simulink model "mpc555rt_io"  (Simulink 6.0)
settings: Solver=FixedStepDiscrete  StartTime=0.0  StopTime=inf  FixedStep=0.01  RelTol=1e-3
PreLoadFcn:
  | RTWConfigurationCB('preloadfcn', bdroot);
undefined symbols (not defined in the file or in its folder): Target_IO, Target_IO_lib5
libraries: mpc555drivers x15, canblocks x8, mpc555toucan x8
CloseFcn:
  | rtwprivate ssgencode ModelCloseRequest mpc555iodemo
settings Model: Creator=The MathWorks Inc.  LastModifiedBy=batserve  ExtModeAutoUpdateStatusClock=off  ProdHWDeviceType=Motorola PowerPC
settings DataIOCC: SaveFormat=StructureWithTime  SignalLoggingName=sigsOut
settings OptimizationCC: BooleanDataType=off  InlineParams=on  InlineInvariantSignals=off  RollThreshold=10  OptimizeModelRefInitCode=on  LifeSpan=1
settings DebuggingCC: CheckExecutionContextPreStartOutputMsg=on  CheckExecutionContextRuntimeOutputMsg=on  SolverPrmCheckMsg=none
settings HardwareCC: ProdEndianess=BigEndian  ProdHWDeviceType=Motorola PowerPC  TargetHWDeviceType=32-bit Generic
settings ModelReferenceCC: UpdateModelReferenceTargets=IfOutOfDate
settings RTWCC: SystemTargetFile=mpc555rt.tlc  TemplateMakefile=mpc555rt.tmf  Description=Embedded Target for Motorola MPC555 (real-time target)  ProcessScript=mpc555rt_make_rtw_hook
settings CodeAppCC: IgnoreCustomStorageClasses=off
settings STFCustomTargetCC: TargetFcnLib=ansi_tfl_tmw.mat  GenFloatMathFcnCalls=ANSI_C  ModelReferenceCompliant=off  CombineOutputUpdateFcns=on  ERTCustomFileBanners=on  SystemTargetFile=mpc555rt.tlc
settings ERTTargetCC: TargetFcnLib=ansi_tfl_tmw.mat  GenFloatMathFcnCalls=ANSI_C  ModelReferenceCompliant=off  SupportContinuousTime=on  SupportNonInlinedSFcns=on  RootIOFormat=Individual Arguments  ERTCustomFileTemplate=example_file_process.tlc  InitialValueSource=Model
settings CustomProperty: DataType=RTWOptions_EnumType__toolbox_rtw_targets_mpc555dk_mpc555dk_mpc555rt_MPC555_OPTIMIZATION_SWITCH  Value=speed
settings EnumStrPairs: String=speed

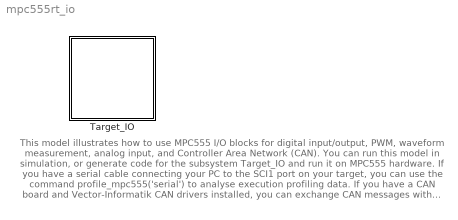
== system mpc555rt_io ==
  note: This model illustrates how to use MPC555 I/O
      | blocks for digital input/output, PWM, waveform
      | measurement, analog input, and Controller Area Network (CAN).
      |
      | You can run this model in simulation, or generate
      | code for the subsystem Target_IO and run it on
      | MPC555 hardware.
      |
      | If you have a serial cable connecting your PC to the SCI1
      | port on your target, you can use the command
      | profile_mpc555('serial') to analyse execution profiling data.
      |
      | If you have a CAN board and Vector-Informatik
      | CAN drivers installed, you can exchange CAN messages
      | with the companion model mpc555rt_iohost.
  Target_IO : Subsystem  InitFcn=|  PropExecContextAcrossSSBoundary=on
      | % START RTW CONFIGURATION CODE %
      | RTWConfigurationCB('rtw_target_initfcn',gcb);
      | % END RTW CONFIGURATION CODE %
      mask Display: image(imread('target_affordance_icon.jpg'),'bottom-right')

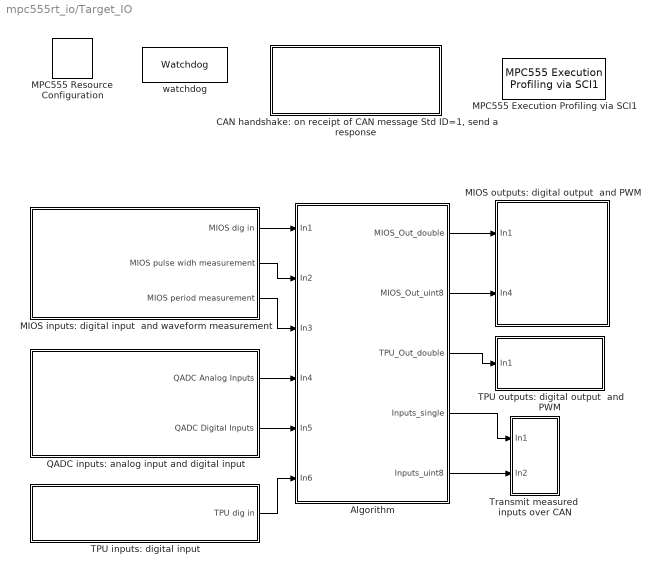
== system mpc555rt_io/Target_IO ==
  Algorithm : Subsystem  PropExecContextAcrossSSBoundary=on
  "CAN handshake: on receipt of CAN message Std ID=1, send a response" : Subsystem  PropExecContextAcrossSSBoundary=on
  MIOS inputs: digital input  and waveform measurement : Subsystem  PropExecContextAcrossSSBoundary=on
  MIOS outputs: digital output  and PWM : Subsystem  PropExecContextAcrossSSBoundary=on
  "MPC555 Resource Configuration " : mpc555drivers/MPC555 Resource Configuration  Tag=RTW CONFIGURATION BLOCK  Priority=-100000  oldParentName=Target_IO_lib5/Target_IO  oldBlockName=|  defaultConfigLibrary=mpc555drivers
      | Target_IO_lib5/Target_IO/MPC555
      | Resource
      | Configuration
  MPC555 Execution Profiling via SCI1 : mpc555drivers/Execution Profiling/MPC555 Execution Profiling via SCI1  t=0.01  execCopyFcn=off
  QADC inputs: analog input and digital input : Subsystem  PropExecContextAcrossSSBoundary=on
  TPU inputs: digital input : Subsystem  PropExecContextAcrossSSBoundary=on
  TPU outputs: digital output  and PWM : Subsystem  PropExecContextAcrossSSBoundary=on
  Transmit measured  inputs over CAN : Subsystem  PropExecContextAcrossSSBoundary=on
  watchdog : mpc555drivers/Watchdog  timeout=0.1
  wires:
  MIOS inputs: digital input  and waveform measurement/1(MIOS dig in) -> Algorithm/1(In1)
  Algorithm/1(MIOS_Out_double) -> MIOS outputs: digital output  and PWM/1(In1)
  MIOS inputs: digital input  and waveform measurement/2(MIOS pulse widh measurement) -> Algorithm/2(In2)
  MIOS inputs: digital input  and waveform measurement/3(MIOS period measurement) -> Algorithm/3(In3)
  QADC inputs: analog input and digital input/1(QADC Analog Inputs) -> Algorithm/4(In4)
  QADC inputs: analog input and digital input/2(QADC Digital Inputs) -> Algorithm/5(In5)
  Algorithm/2(MIOS_Out_uint8) -> MIOS outputs: digital output  and PWM/2(In4)
  Algorithm/3(TPU_Out_double) -> TPU outputs: digital output  and PWM/1(In1)
  TPU inputs: digital input/1(TPU dig in) -> Algorithm/6(In6)
  Algorithm/4(Inputs_single) -> Transmit measured  inputs over CAN/1(In1)
  Algorithm/5(Inputs_uint8) -> Transmit measured  inputs over CAN/2(In2)

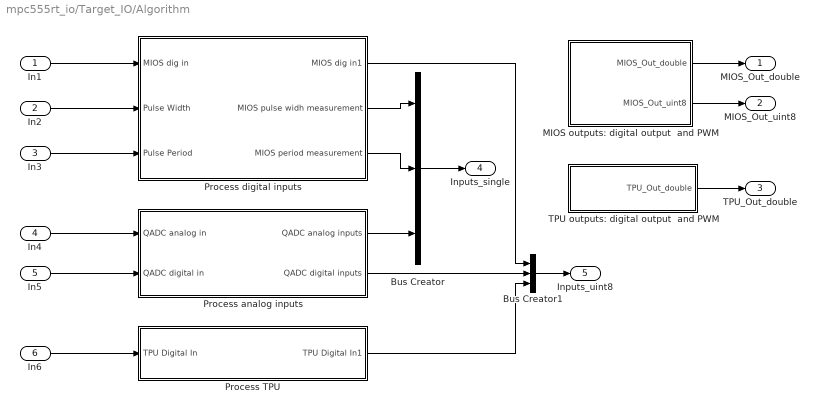
== system mpc555rt_io/Target_IO/Algorithm ==
  In1 : Inport  Port=1  LatchInput=off
  In2 : Inport  Port=2  LatchInput=off
  In3 : Inport  Port=3  LatchInput=off
  In4 : Inport  Port=4  LatchInput=off
  In5 : Inport  Port=5  LatchInput=off
  In6 : Inport  Port=6  LatchInput=off
  Bus Creator : BusCreator  DialogController=Simulink.DDGSource_Bus  Inputs=3
  Bus Creator1 : BusCreator  DialogController=Simulink.DDGSource_Bus  Inputs=3
  MIOS outputs: digital output  and PWM : Subsystem  PropExecContextAcrossSSBoundary=on
  Process TPU : Subsystem  PropExecContextAcrossSSBoundary=on
  Process analog inputs : Subsystem  PropExecContextAcrossSSBoundary=on
  Process digital inputs : Subsystem  PropExecContextAcrossSSBoundary=on
  TPU outputs: digital output  and PWM : Subsystem  PropExecContextAcrossSSBoundary=on
  MIOS_Out_double : Outport
  MIOS_Out_uint8 : Outport  Port=2
  TPU_Out_double : Outport  Port=3
  Inputs_single : Outport  Port=4
  Inputs_uint8 : Outport  Port=5
  wires:
  Process digital inputs/1(MIOS dig in1) -> Bus Creator1/1
  Process digital inputs/2(MIOS pulse widh measurement) -> Bus Creator/1
  Process digital inputs/3(MIOS period measurement) -> Bus Creator/2
  Process analog inputs/1(QADC analog inputs) -> Bus Creator/3
  In1/1 -> Process digital inputs/1(MIOS dig in)
  MIOS outputs: digital output  and PWM/1(MIOS_Out_double) -> MIOS_Out_double/1
  In2/1 -> Process digital inputs/2(Pulse Width)
  In3/1 -> Process digital inputs/3(Pulse Period)
  MIOS outputs: digital output  and PWM/2(MIOS_Out_uint8) -> MIOS_Out_uint8/1
  In4/1 -> Process analog inputs/1(QADC analog in)
  In5/1 -> Process analog inputs/2(QADC digital in)
  TPU outputs: digital output  and PWM/1(TPU_Out_double) -> TPU_Out_double/1
  Process analog inputs/2(QADC digital inputs) -> Bus Creator1/2
  Process TPU/1(TPU Digital In1) -> Bus Creator1/3
  Bus Creator/1 -> Inputs_single/1
  Bus Creator1/1 -> Inputs_uint8/1
  In6/1 -> Process TPU/1(TPU Digital In)

== system mpc555rt_io/Target_IO/CAN handshake: on receipt of CAN message Std ID=1, send a response ==
  note: HANDSHAKE TEST
  note: On receipt of CAN message with standard ID=1 a response message with standard ID=2 is constructed from the data in the received message.
      | If you have appropriate CAN hardware on your PC, you can use the corresponding host-side model to transmit the message with ID=1.
  Real Time Transmit  Std ID = 2 : Subsystem  TreatAsAtomicUnit=on  PropExecContextAcrossSSBoundary=on
  TouCAN Receive1 : mpc555toucan/TouCAN Receive  module=A  ids=1  notification_type=Function Call Outport  auto_select_buffer=on  bufferids=3  use_queue=off  queue_length=3  message_type=Standard (11-bit identifier)  t=1
  wires:
  TouCAN Receive1/1 -> Real Time Transmit  Std ID = 2/Trigger
  TouCAN Receive1/2 -> Real Time Transmit  Std ID = 2/1(Message)

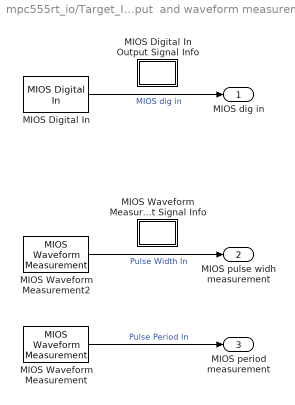
== system mpc555rt_io/Target_IO/MIOS inputs: digital input  and waveform measurement ==
  MIOS Digital In : mpc555drivers/Modular Input//Output System (MIOS1)/MIOS Digital In  bits=[8 9 10 11 12 13 14 15]  t=0.1  enablePassThru=off
  MIOS Digital In Output Signal Info : Subsystem  Orientation=left  PropExecContextAcrossSSBoundary=on
      mask Display: disp('Info')
  MIOS Waveform Measurement : mpc555drivers/Modular Input//Output System (MIOS1)/MIOS Waveform Measurement  module=12  operation=Pulse period  bsl=Counter Bus 6 (CB6)  range=[ 0.0002048 , 13.4218 ]  t=0.1  edpol=off  fren=off  enablePassThru=off
  MIOS Waveform Measurement Output Signal Info : Subsystem  Orientation=left  PropExecContextAcrossSSBoundary=on
      mask Display: disp('Info')
  MIOS Waveform Measurement2 : mpc555drivers/Modular Input//Output System (MIOS1)/MIOS Waveform Measurement  module=11  operation=Pulse width  bsl=Counter Bus 6 (CB6)  range=[ 0.0002048 , 13.4218 ]  t=0.1  edpol=off  fren=off  enablePassThru=off
  MIOS dig in : Outport
  MIOS pulse widh measurement : Outport  Port=2
  MIOS period measurement : Outport  Port=3
  wires:
  MIOS Digital In/1 -> MIOS dig in/1  "MIOS dig in"
  MIOS Waveform Measurement/1 -> MIOS period measurement/1  "Pulse Period In"
  MIOS Waveform Measurement2/1 -> MIOS pulse widh measurement/1  "Pulse Width In"

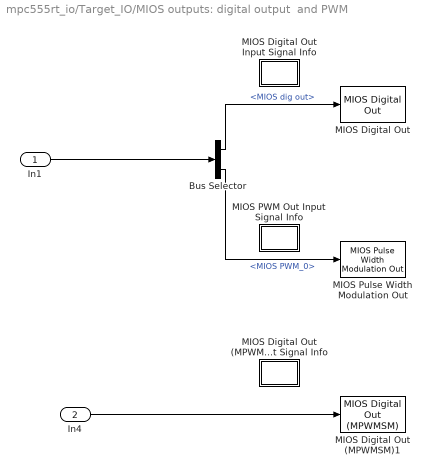
== system mpc555rt_io/Target_IO/MIOS outputs: digital output  and PWM ==
  In1 : Inport  Port=1  LatchInput=off
  In4 : Inport  Port=2  LatchInput=off
  Bus Selector : BusSelector  DialogController=Simulink.DDGSource_Bus  OutputSignals=MIOS dig out,MIOS PWM_0
  MIOS Digital Out : mpc555drivers/Modular Input//Output System (MIOS1)/MIOS Digital Out  bits=[0 1 2 3 4 5 6 7]  init=0  t=-1  enablePassThru=off
  MIOS Digital Out (MPWMSM)1 : mpc555drivers/Modular Input//Output System (MIOS1)/MIOS Digital Out (MPWMSM)  Priority=2  module=17  init=0  t=-1  enablePassThru=off
  MIOS Digital Out Input Signal Info : Subsystem  Orientation=left  PropExecContextAcrossSSBoundary=on
      mask Display: disp('Info')
  MIOS Digital Out (MPWMSM) Input Signal Info : Subsystem  Orientation=left  PropExecContextAcrossSSBoundary=on
      mask Display: disp('Info')
  MIOS PWM Out Input Signal Info : Subsystem  Orientation=left  PropExecContextAcrossSSBoundary=on
      mask Display: disp('Info')
  MIOS Pulse Width Modulation Out : mpc555drivers/Modular Input//Output System (MIOS1)/MIOS Pulse Width Modulation Out  Priority=2  module=0  timing_settings=off  period=0.01  initpw=0.5  cp=255  pp=12500  t=-1  pol=on  trsp=on  fren=off  enablePassThru=off
  wires:
  Bus Selector/1 -> MIOS Digital Out/1  "<MIOS dig out>"
  Bus Selector/2 -> MIOS Pulse Width Modulation Out/1  "<MIOS PWM_0>"
  In4/1 -> MIOS Digital Out (MPWMSM)1/1
  In1/1 -> Bus Selector/1

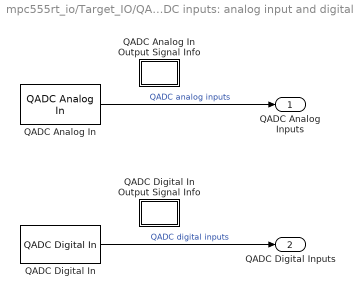
== system mpc555rt_io/Target_IO/QADC inputs: analog input and digital input ==
  QADC Analog In : mpc555drivers/Queued Analog-To-Digital Converter Module-64/QADC Analog In  module=B  channels=[0 1]  justification=Right-justified (unsigned)  t=0.1  enablePassThru=off
  QADC Analog In Output Signal Info : Subsystem  Orientation=left  PropExecContextAcrossSSBoundary=on
      mask Display: disp('Info')
  QADC Digital In : mpc555drivers/Queued Analog-To-Digital Converter Module-64/QADC Digital In  module=A  port=B  bits=[0 1 2 3]  t=1  enablePassThru=off
  QADC Digital In Output Signal Info : Subsystem  Orientation=left  PropExecContextAcrossSSBoundary=on
      mask Display: disp('Info')
  QADC Analog Inputs : Outport
  QADC Digital Inputs : Outport  Port=2
  wires:
  QADC Analog In/1 -> QADC Analog Inputs/1  "QADC analog inputs"
  QADC Digital In/1 -> QADC Digital Inputs/1  "QADC digital inputs"

== system mpc555rt_io/Target_IO/TPU inputs: digital input ==
  TPU Digital In Output Signal Info : Subsystem  Orientation=left  PropExecContextAcrossSSBoundary=on
      mask Display: disp('Info')
  TPU3 Digital In : mpc555drivers/Time Processor Unit (TPU3)/TPU3 Digital In  module=B  channel=0  channel_priority=Low  sampleTime=0.1  enablePassThru=off
  TPU dig in : Outport
  wires:
  TPU3 Digital In/1 -> TPU dig in/1  "TPU dig in"

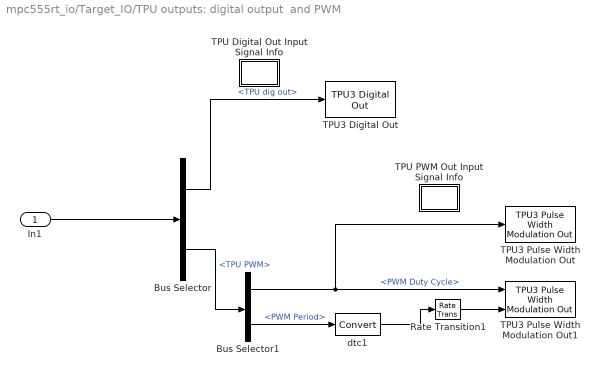
== system mpc555rt_io/Target_IO/TPU outputs: digital output  and PWM ==
  In1 : Inport  Port=1  LatchInput=off
  Bus Selector : BusSelector  DialogController=Simulink.DDGSource_Bus  OutputSignals=TPU dig out,TPU PWM
  Bus Selector1 : BusSelector  DialogController=Simulink.DDGSource_Bus  OutputSignals=PWM Duty Cycle,PWM Period
  Rate Transition1 : RateTransition
  TPU Digital Out Input Signal Info : Subsystem  Orientation=left  PropExecContextAcrossSSBoundary=on
      mask Display: disp('Info')
  TPU PWM Out Input Signal Info : Subsystem  Orientation=left  PropExecContextAcrossSSBoundary=on
      mask Display: disp('Info')
  TPU3 Digital Out : mpc555drivers/Time Processor Unit (TPU3)/TPU3 Digital Out  module=A  channel=0  channel_priority=Medium  sampleTime=-1  enablePassThru=off
  TPU3 Pulse Width Modulation Out : mpc555drivers/Time Processor Unit (TPU3)/TPU3 Pulse Width Modulation Out  module=A  channel=1  channel_priority=Medium  block_period=off  timing_settings=off  ideal_period=0.02  PWMPER=12500  actual_period=0.02  sampleTime=-1  enablePassThru=off
  TPU3 Pulse Width Modulation Out1 : mpc555drivers/Time Processor Unit (TPU3)/TPU3 Pulse Width Modulation Out  module=B  channel=1  channel_priority=Medium  block_period=on  timing_settings=off  ideal_period=0.02  PWMPER=12500  actual_period=0.02  sampleTime=0.01  enablePassThru=off
  dtc1 : DataTypeConversion  OutDataTypeMode=uint16  SaturateOnIntegerOverflow=on  RndMeth=Zero
  wires:
  Bus Selector/2 -> Bus Selector1/1  "<TPU PWM>"
  Bus Selector/1 -> TPU3 Digital Out/1  "<TPU dig out>"
  Bus Selector1/1 -> TPU3 Pulse Width Modulation Out1/1, TPU3 Pulse Width Modulation Out/1  "<PWM Duty Cycle>"
  Bus Selector1/2 -> dtc1/1  "<PWM Period>"
  dtc1/1 -> Rate Transition1/1
  Rate Transition1/1 -> TPU3 Pulse Width Modulation Out1/2
  In1/1 -> Bus Selector/1

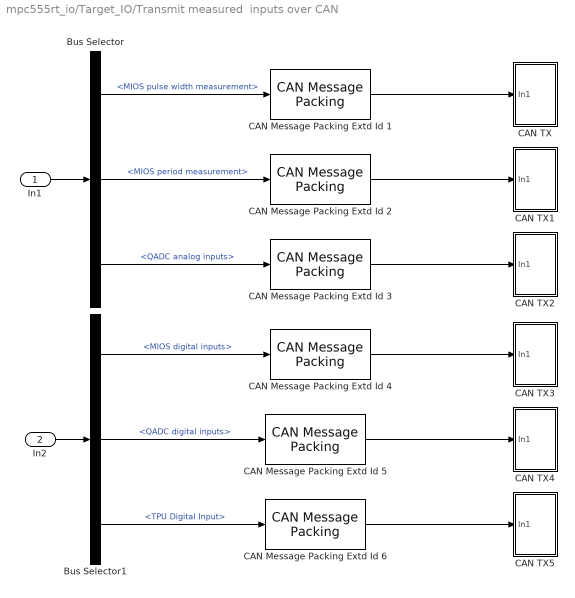
== system mpc555rt_io/Target_IO/Transmit measured  inputs over CAN ==
  In1 : Inport  Port=1  LatchInput=off
  In2 : Inport  Port=2  LatchInput=off
  Bus Selector : BusSelector  DialogController=Simulink.DDGSource_Bus  OutputSignals=MIOS pulse width measurement,MIOS period measurement,QADC analog inputs
  Bus Selector1 : BusSelector  DialogController=Simulink.DDGSource_Bus  OutputSignals=MIOS digital inputs,QADC digital inputs,TPU Digital Input
  CAN Message Packing Extd Id 1 : canblocks/CAN Message Packing  id=1  message_type=Extended (29-bit identifier)  endian=Big Endian (Motorola)
  CAN Message Packing Extd Id 2 : canblocks/CAN Message Packing  id=2  message_type=Extended (29-bit identifier)  endian=Big Endian (Motorola)
  CAN Message Packing Extd Id 3 : canblocks/CAN Message Packing  id=3  message_type=Extended (29-bit identifier)  endian=Big Endian (Motorola)
  CAN Message Packing Extd Id 4 : canblocks/CAN Message Packing  id=4  message_type=Extended (29-bit identifier)  endian=Big Endian (Motorola)
  CAN Message Packing Extd Id 5 : canblocks/CAN Message Packing  id=5  message_type=Extended (29-bit identifier)  endian=Big Endian (Motorola)
  CAN Message Packing Extd Id 6 : canblocks/CAN Message Packing  id=6  message_type=Extended (29-bit identifier)  endian=Big Endian (Motorola)
  CAN TX : Subsystem  PropExecContextAcrossSSBoundary=on
  CAN TX1 : Subsystem  PropExecContextAcrossSSBoundary=on
  CAN TX2 : Subsystem  PropExecContextAcrossSSBoundary=on
  CAN TX3 : Subsystem  PropExecContextAcrossSSBoundary=on
  CAN TX4 : Subsystem  PropExecContextAcrossSSBoundary=on
  CAN TX5 : Subsystem  PropExecContextAcrossSSBoundary=on
  wires:
  In1/1 -> Bus Selector/1
  In2/1 -> Bus Selector1/1
  Bus Selector/1 -> CAN Message Packing Extd Id 1/1  "<MIOS pulse width measurement>"
  Bus Selector/2 -> CAN Message Packing Extd Id 2/1  "<MIOS period measurement>"
  Bus Selector/3 -> CAN Message Packing Extd Id 3/1  "<QADC analog inputs>"
  Bus Selector1/1 -> CAN Message Packing Extd Id 4/1  "<MIOS digital inputs>"
  Bus Selector1/2 -> CAN Message Packing Extd Id 5/1  "<QADC digital inputs>"
  Bus Selector1/3 -> CAN Message Packing Extd Id 6/1  "<TPU Digital Input>"
  CAN Message Packing Extd Id 1/1 -> CAN TX/1(In1)
  CAN Message Packing Extd Id 2/1 -> CAN TX1/1(In1)
  CAN Message Packing Extd Id 3/1 -> CAN TX2/1(In1)
  CAN Message Packing Extd Id 4/1 -> CAN TX3/1(In1)
  CAN Message Packing Extd Id 5/1 -> CAN TX4/1(In1)
  CAN Message Packing Extd Id 6/1 -> CAN TX5/1(In1)

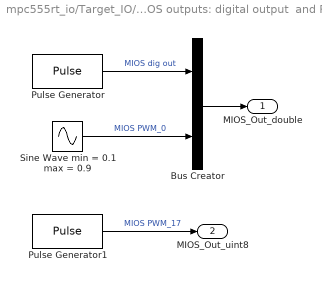
== system mpc555rt_io/Target_IO/Algorithm/MIOS outputs: digital output  and PWM ==
  Bus Creator : BusCreator  DialogController=Simulink.DDGSource_Bus  Inputs=2
  Pulse Generator : DiscretePulseGenerator  Amplitude=ones(1,8)  Period=15  PhaseDelay=[0 1 2 3 4 5 6 7]  SampleTime=0.1
  Pulse Generator1 : DiscretePulseGenerator  Amplitude=uint8(1)  Period=5  SampleTime=0.01
  Sine Wave min = 0.1 max = 0.9 : Sin  SineType=Sample based  Amplitude=0.4  Bias=0.5  Samples=5000  SampleTime=0.01
  MIOS_Out_double : Outport
  MIOS_Out_uint8 : Outport  Port=2
  wires:
  Pulse Generator/1 -> Bus Creator/1  "MIOS dig out"
  Sine Wave min = 0.1 max = 0.9/1 -> Bus Creator/2  "MIOS PWM_0"
  Pulse Generator1/1 -> MIOS_Out_uint8/1  "MIOS PWM_17"
  Bus Creator/1 -> MIOS_Out_double/1

== system mpc555rt_io/Target_IO/Algorithm/Process TPU ==
  TPU Digital In : Inport  Port=1  LatchInput=off
  Data Type Conversion3 : DataTypeConversion  OutDataTypeMode=uint8  SaturateOnIntegerOverflow=on  RndMeth=Zero
  TPU Digital In1 : Outport
  wires:
  TPU Digital In/1 -> Data Type Conversion3/1
  Data Type Conversion3/1 -> TPU Digital In1/1  "TPU Digital Input"

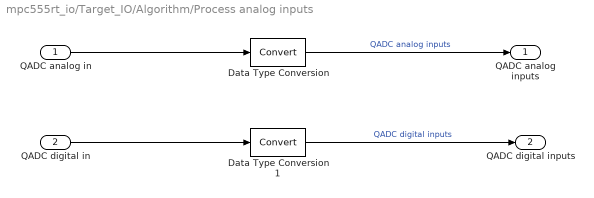
== system mpc555rt_io/Target_IO/Algorithm/Process analog inputs ==
  QADC analog in : Inport  Port=1  LatchInput=off
  QADC digital in : Inport  Port=2  LatchInput=off
  Data Type Conversion : DataTypeConversion  OutDataTypeMode=single  SaturateOnIntegerOverflow=on  RndMeth=Zero
  Data Type Conversion1 : DataTypeConversion  OutDataTypeMode=uint8  SaturateOnIntegerOverflow=on  RndMeth=Zero
  QADC analog inputs : Outport
  QADC digital inputs : Outport  Port=2
  wires:
  Data Type Conversion/1 -> QADC analog inputs/1  "QADC analog inputs"
  QADC digital in/1 -> Data Type Conversion1/1
  QADC analog in/1 -> Data Type Conversion/1
  Data Type Conversion1/1 -> QADC digital inputs/1  "QADC digital inputs"

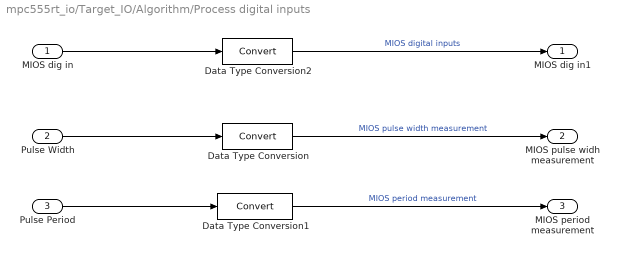
== system mpc555rt_io/Target_IO/Algorithm/Process digital inputs ==
  MIOS dig in : Inport  Port=1  LatchInput=off
  Pulse Width : Inport  Port=2  LatchInput=off
  Pulse Period : Inport  Port=3  LatchInput=off
  Data Type Conversion : DataTypeConversion  OutDataTypeMode=single  SaturateOnIntegerOverflow=on  RndMeth=Zero
  Data Type Conversion1 : DataTypeConversion  OutDataTypeMode=single  SaturateOnIntegerOverflow=on  RndMeth=Zero
  Data Type Conversion2 : DataTypeConversion  OutDataTypeMode=uint8  SaturateOnIntegerOverflow=on  RndMeth=Zero
  MIOS dig in1 : Outport
  MIOS pulse widh measurement : Outport  Port=2
  MIOS period measurement : Outport  Port=3
  wires:
  Data Type Conversion/1 -> MIOS pulse widh measurement/1  "MIOS pulse width measurement"
  Data Type Conversion1/1 -> MIOS period measurement/1  "MIOS period measurement"
  Data Type Conversion2/1 -> MIOS dig in1/1  "MIOS digital inputs"
  Pulse Width/1 -> Data Type Conversion/1
  Pulse Period/1 -> Data Type Conversion1/1
  MIOS dig in/1 -> Data Type Conversion2/1

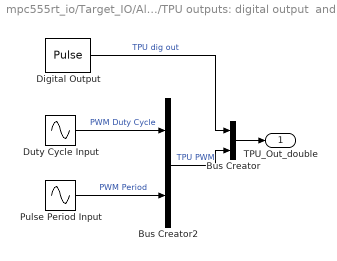
== system mpc555rt_io/Target_IO/Algorithm/TPU outputs: digital output  and PWM ==
  Bus Creator : BusCreator  DialogController=Simulink.DDGSource_Bus  Inputs=2
  Bus Creator2 : BusCreator  DialogController=Simulink.DDGSource_Bus  Inputs=2
  Digital Output : DiscretePulseGenerator
  Duty Cycle Input : Sin  SineType=Sample based  Amplitude=.5  Bias=.5  Samples=200  SampleTime=0.01
  Pulse Period Input : Sin  SineType=Sample based  Amplitude=10000  Bias=20000  Samples=100  SampleTime=0.5
  TPU_Out_double : Outport
  wires:
  Bus Creator2/1 -> Bus Creator/2  "TPU PWM"
  Digital Output/1 -> Bus Creator/1  "TPU dig out"
  Duty Cycle Input/1 -> Bus Creator2/1  "PWM Duty Cycle"
  Pulse Period Input/1 -> Bus Creator2/2  "PWM Period"
  Bus Creator/1 -> TPU_Out_double/1

== system mpc555rt_io/Target_IO/CAN handshake: on receipt of CAN message Std ID=1, send a response/Real Time Transmit  Std ID = 2 ==
  Message : Inport  Port=1  LatchInput=off
  function : TriggerPort  TriggerType=function-call
  CAN Message Packing Std Id = 2 : canblocks/CAN Message Packing  id=2  message_type=Standard (11-bit identifier)  endian=Big Endian (Motorola)
  CAN Message Unpacking : canblocks/CAN Message Unpacking/CAN Message Unpacking  showData=on  showID=off  showLength=off  endian=Little Endian (Intel)
  CAN TX : Subsystem  PropExecContextAcrossSSBoundary=on
  Signal Specification : SignalSpecification  Dimensions=8  DataType=uint8
  wires:
  Signal Specification/1 -> CAN Message Packing Std Id = 2/1
  CAN Message Unpacking/1 -> Signal Specification/1
  Message/1 -> CAN Message Unpacking/1
  CAN Message Packing Std Id = 2/1 -> CAN TX/1(In1)

== system mpc555rt_io/Target_IO/MIOS inputs: digital input  and waveform measurement/MIOS Digital In Output Signal Info ==
  note: The output is a boolean, either true or false

== system mpc555rt_io/Target_IO/MIOS inputs: digital input  and waveform measurement/MIOS Waveform Measurement Output Signal Info ==
  note: The output signal is the pulse width or pulse period, measured
      | in seconds. The valid range is determined by the dialog settings
      | in the MIOS Waveform Measurement block and the corresponding
      | settings in the MPC555 Resource Configuration block. The allowed
      | datatype for this signal is either double or single.

== system mpc555rt_io/Target_IO/MIOS outputs: digital output  and PWM/MIOS Digital Out Input Signal Info ==
  note: The input signal is interpreted as either true or false

== system mpc555rt_io/Target_IO/MIOS outputs: digital output  and PWM/MIOS Digital Out (MPWMSM) Input Signal Info ==
  note: The input signal is interpreted as either true or false

== system mpc555rt_io/Target_IO/MIOS outputs: digital output  and PWM/MIOS PWM Out Input Signal Info ==
  note: The input signal must be scaled in the range 0 to 1, the datatype
      | may be either double or single.

== system mpc555rt_io/Target_IO/QADC inputs: analog input and digital input/QADC Analog In Output Signal Info ==
  note: The output signal is either a uint16 or an int16 depending on whether signed
      | or unsigned is selected in the mask dialog. While the value is provided
      | as a 16 bit word, the actual resolution is only 10 bits. The 10 bit ADC
      | reading is either right or left justified within the 16 bit word depending
      | on the option selected in the mask dialog.

== system mpc555rt_io/Target_IO/QADC inputs: analog input and digital input/QADC Digital In Output Signal Info ==
  note: The output signal is either true or false

== system mpc555rt_io/Target_IO/TPU inputs: digital input/TPU Digital In Output Signal Info ==
  note: The output is a boolean, either true or false

== system mpc555rt_io/Target_IO/TPU outputs: digital output  and PWM/TPU Digital Out Input Signal Info ==
  note: The input signal is interpreted as either true or false

== system mpc555rt_io/Target_IO/TPU outputs: digital output  and PWM/TPU PWM Out Input Signal Info ==
  note: Input signal 1, the Duty Cycle input, must be scaled in the range 0 to 1,
      | the datatype may be either double or single.
      |
      | Input signal 2 (optional), the Period Register input, must be a uint16 value.

== system mpc555rt_io/Target_IO/Transmit measured  inputs over CAN/CAN TX ==
  In1 : Inport  Port=1  LatchInput=off
  TouCAN Transmit : mpc555toucan/TouCAN Transmit  module=A  tx_mode=Queued transmission with shared buffer  fifo_queue_length=8  bufferids=0  t=-1  enablePassThru=off
  wires:
  In1/1 -> TouCAN Transmit/1

== system mpc555rt_io/Target_IO/Transmit measured  inputs over CAN/CAN TX1 ==
  In1 : Inport  Port=1  LatchInput=off
  TouCAN Transmit1 : mpc555toucan/TouCAN Transmit  module=A  tx_mode=Queued transmission with shared buffer  fifo_queue_length=8  bufferids=0  t=-1  enablePassThru=off
  wires:
  In1/1 -> TouCAN Transmit1/1

== system mpc555rt_io/Target_IO/Transmit measured  inputs over CAN/CAN TX2 ==
  In1 : Inport  Port=1  LatchInput=off
  TouCAN Transmit2 : mpc555toucan/TouCAN Transmit  module=A  tx_mode=Queued transmission with shared buffer  fifo_queue_length=8  bufferids=0  t=-1  enablePassThru=off
  wires:
  In1/1 -> TouCAN Transmit2/1

== system mpc555rt_io/Target_IO/Transmit measured  inputs over CAN/CAN TX3 ==
  In1 : Inport  Port=1  LatchInput=off
  TouCAN Transmit3 : mpc555toucan/TouCAN Transmit  module=A  tx_mode=Queued transmission with shared buffer  fifo_queue_length=8  bufferids=0  t=-1  enablePassThru=off
  wires:
  In1/1 -> TouCAN Transmit3/1

== system mpc555rt_io/Target_IO/Transmit measured  inputs over CAN/CAN TX4 ==
  In1 : Inport  Port=1  LatchInput=off
  TouCAN Transmit4 : mpc555toucan/TouCAN Transmit  module=A  tx_mode=Queued transmission with shared buffer  fifo_queue_length=8  bufferids=0  t=-1  enablePassThru=off
  wires:
  In1/1 -> TouCAN Transmit4/1

== system mpc555rt_io/Target_IO/Transmit measured  inputs over CAN/CAN TX5 ==
  In1 : Inport  Port=1  LatchInput=off
  TouCAN Transmit5 : mpc555toucan/TouCAN Transmit  module=A  tx_mode=Queued transmission with shared buffer  fifo_queue_length=8  bufferids=0  t=-1  enablePassThru=off
  wires:
  In1/1 -> TouCAN Transmit5/1

== system mpc555rt_io/Target_IO/CAN handshake: on receipt of CAN message Std ID=1, send a response/Real Time Transmit  Std ID = 2/CAN TX ==
  In1 : Inport  Port=1  LatchInput=off
  TouCAN Transmit : mpc555toucan/TouCAN Transmit  module=A  tx_mode=Queued transmission with shared buffer  fifo_queue_length=8  bufferids=0  t=-1  enablePassThru=off
  wires:
  In1/1 -> TouCAN Transmit/1
